simulink library "Crazyflie_Library"  (R2019a)
settings: Solver=VariableStepAuto  StartTime=0.0  StopTime=10.0  RelTol=1e-3
values from neighbouring files (symbols this model uses):
  DeePC_param = evalin('base', 'DeePC_param')    [DeePC_Optimizer_osqp.m]
  param = evalin('base', 'param')    [DeePC_Optimizer_osqp.m]    (also in DeePC_main.m = load_crazyflie_parameters(i_aux))
undefined symbols (not defined in the file or in its folder): DiscIntNeverNeededParam
libraries: simulink x3, $bdroot x3
(part 2 of 2)

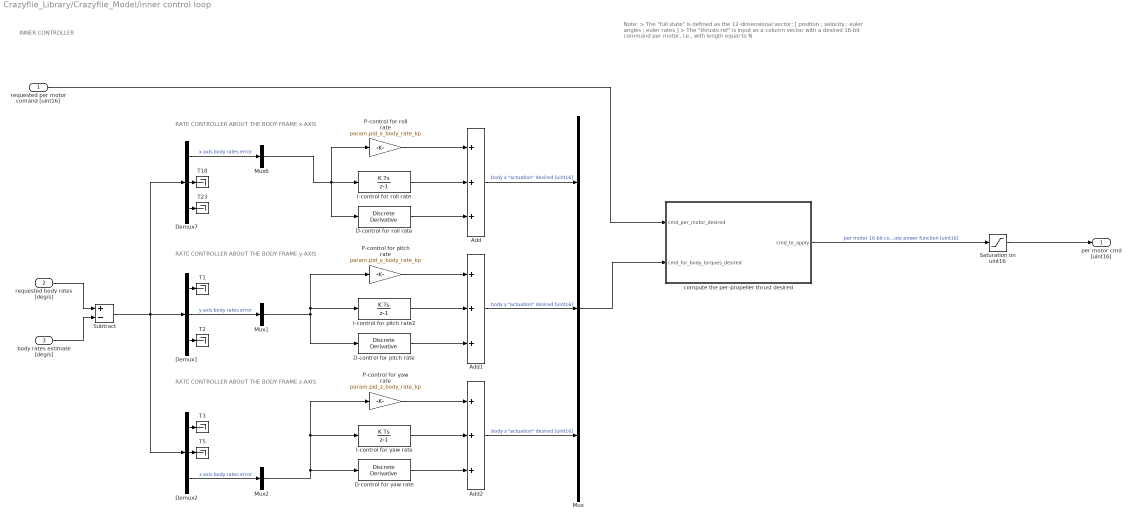
== system Crazyflie_Library/Crazyflie_Model/inner control loop ==
  note: RATE CONTROLLER ABOUT THE BODY FRAME z-AXIS
  note: RATE CONTROLLER ABOUT THE BODY FRAME y-AXIS
  note: RATE CONTROLLER ABOUT THE BODY FRAME x-AXIS
  note: INNER CONTROLLER
  note: Note:
      | > The "full state" is defined as the 12-dimensional vector:
      | [ position ; velocity ; euler angles ; euler rates ]
      | > The "thrusts ref" is input as a column vector with a desired
      | 16-bit command per motor, i.e., with length equal to N
  requested per motor comand [uint16] : Inport
  requested body rates [deg/s] : Inport  Port=2
  body rates estimate [deg/s] : Inport  Port=3
  Add : Sum  Inputs=+++
  Add1 : Sum  Inputs=+++
  Add2 : Sum  Inputs=+++
  D-control for pitch rate : simulink/Discrete/Discrete Derivative  gainval=param.pid_y_body_rate_kd  ICPrevScaledInput=0.0  OutMin=[]  OutMax=[]  OutDataType=fixdt(1, 16)  OutScaling=2^-10  DoSatur=off
  D-control for roll rate : simulink/Discrete/Discrete Derivative  gainval=param.pid_x_body_rate_kd  ICPrevScaledInput=0.0  OutMin=[]  OutMax=[]  OutDataType=fixdt(1, 16)  OutScaling=2^-10  DoSatur=off
  D-control for yaw rate : simulink/Discrete/Discrete Derivative  gainval=param.pid_z_body_rate_kd  ICPrevScaledInput=0.0  OutMin=[]  OutMax=[]  OutDataType=fixdt(1, 16)  OutScaling=2^-10  DoSatur=off
  Demux1 : Demux  Outputs=3
  Demux2 : Demux  Outputs=3
  Demux7 : Demux  Outputs=3
  I-control for pitch rate2 : DiscreteIntegrator  gainval=param.pid_y_body_rate_ki  SampleTime=-1  LimitOutput=on  UpperSaturationLimit=param.pid_y_body_rate_integrator_limit  LowerSaturationLimit=-param.pid_y_body_rate_integrator_limit  ICPrevOutput=DiscIntNeverNeededParam  ICPrevScaledInput=DiscIntNeverNeededParam
  I-control for roll rate : DiscreteIntegrator  gainval=param.pid_x_body_rate_ki  SampleTime=-1  LimitOutput=on  UpperSaturationLimit=param.pid_x_body_rate_integrator_limit  LowerSaturationLimit=-param.pid_x_body_rate_integrator_limit  ICPrevOutput=DiscIntNeverNeededParam  ICPrevScaledInput=DiscIntNeverNeededParam
  I-control for yaw rate : DiscreteIntegrator  gainval=param.pid_z_body_rate_ki  SampleTime=-1  LimitOutput=on  UpperSaturationLimit=param.pid_x_body_rate_integrator_limit  LowerSaturationLimit=-param.pid_x_body_rate_integrator_limit  ICPrevOutput=DiscIntNeverNeededParam  ICPrevScaledInput=DiscIntNeverNeededParam
  Mux : Mux  Inputs=3
  Mux1 : Mux  Inputs=1
  Mux2 : Mux  Inputs=1
  Mux6 : Mux  Inputs=1
  P-control for pitch rate : Gain  Gain=param.pid_y_body_rate_kp
  P-control for roll rate : Gain  Gain=param.pid_x_body_rate_kp
  P-control for yaw rate : Gain  Gain=param.pid_z_body_rate_kp
  Saturation on uint16 : Saturate  UpperLimit=param.cmd_max  LowerLimit=param.cmd_min  ZeroCross=off
  Subtract : Sum  Inputs=+-
  T{1..3,5,18,23} (6 alike) : Terminator
  compute the per-propeller thrust desired : MATLAB Function  TreatAsAtomicUnit=on
  per motor cmd [uint16] : Outport
  wires:
  compute the per-propeller thrust desired/1(cmd_to_apply) -> Saturation on uint16/1  "per motor 16-bit command after distribute power function [uint16]"
  body rates estimate [deg/s]/1 -> Subtract/2
  requested per motor comand [uint16]/1 -> compute the per-propeller thrust desired/1(cmd_per_motor_desired)
  requested body rates [deg/s]/1 -> Subtract/1
  Add/1 -> Mux/1  "body x \"actuation\" desired [uint16]"
  Add1/1 -> Mux/2  "body y \"actuation\" desired [uint16]"
  Add2/1 -> Mux/3  "body z \"actuation\" desired [uint16]"
  Subtract/1 -> Demux2/1, Demux1/1, Demux7/1
  Mux/1 -> compute the per-propeller thrust desired/2(cmd_for_body_torques_desired)
  Saturation on uint16/1 -> per motor cmd [uint16]/1
  Demux7/2 -> T18/1
  Mux6/1 -> P-control for roll rate/1, I-control for roll rate/1, D-control for roll rate/1
  Demux7/3 -> T23/1
  Demux7/1 -> Mux6/1  "x axis body rates error"
  Demux1/2 -> Mux1/1  "y axis body rates error"
  Demux1/3 -> T2/1
  Demux1/1 -> T1/1
  Demux2/3 -> Mux2/1  "z axis body rates error"
  Demux2/1 -> T3/1
  Mux2/1 -> I-control for yaw rate/1, P-control for yaw rate/1, D-control for yaw rate/1
  Demux2/2 -> T5/1
  P-control for roll rate/1 -> Add/1
  I-control for roll rate/1 -> Add/2
  D-control for roll rate/1 -> Add/3
  P-control for pitch rate/1 -> Add1/1
  I-control for pitch rate2/1 -> Add1/2
  D-control for pitch rate/1 -> Add1/3
  Mux1/1 -> D-control for pitch rate/1, P-control for pitch rate/1, I-control for pitch rate2/1
  D-control for yaw rate/1 -> Add2/3
  P-control for yaw rate/1 -> Add2/1
  I-control for yaw rate/1 -> Add2/2

== system Crazyflie_Library/Crazyflie_Model/N-rotor vehicle model/Full equations of motions implemented in one shot ==
  thrusts [N] : Inport
  Body rates friction matrix : Constant  Value=param.nrotor_vehicle_body_rates_friction
  Integrator5 : Integrator  InitialCondition=param.nrotor_initial_condition
  Inverse of J : Constant  Value=param.nrotor_vehicle_inertia_inverse
  Matrix describing the vehicle layout : Constant  Value=param.nrotor_vehicle_layout_true
  "Moment of inertia matrix, J" : Constant  Value=param.nrotor_vehicle_inertia
  Position friction matrix : Constant  Value=param.nrotor_vehicle_position_friction
  The full equations of motion implemented with one function : MATLAB Function  TreatAsAtomicUnit=on
  graviational constant : Constant  Value=param.g
  vehicle's mass : Constant  Value=param.nrotor_vehicle_mass_true
  full state : Outport
  body rates : Outport  Port=2
  body accellerations : Outport  Port=3
  wires:
  The full equations of motion implemented with one function/1(full_state_dot) -> Integrator5/1  "full_state_dot"
  Matrix describing the vehicle layout/1 -> The full equations of motion implemented with one function/5(layout)
  The full equations of motion implemented with one function/3(body_accel) -> body accellerations/1
  graviational constant/1 -> The full equations of motion implemented with one function/1(g)
  thrusts [N]/1 -> The full equations of motion implemented with one function/8(thrusts)
  The full equations of motion implemented with one function/2(body_rates) -> body rates/1
  Integrator5/1 -> full state/1, The full equations of motion implemented with one function/9(full_state)  "full_state"
  Inverse of J/1 -> The full equations of motion implemented with one function/4(J_inv)
  vehicle's mass/1 -> The full equations of motion implemented with one function/2(m)
  "Moment of inertia matrix, J"/1 -> The full equations of motion implemented with one function/3(J)
  Position friction matrix/1 -> The full equations of motion implemented with one function/6(pos_fric)
  Body rates friction matrix/1 -> The full equations of motion implemented with one function/7(w_fric)

== system Crazyflie_Library/Crazyflie_Model/N-rotor vehicle model/convert motor comand to thrust ==
  note: CONVERT MOTOR COMMAND AS uint16 VALUE TO THRUST IN NEWTONS
      | > Apply the following equation:
      | thust [N] = nrotor_vehicle_thrust_max * ( cmd_2_newtons_conversion_quadratic_coefficient * cmd^2 + cmd_2_newtons_conversion_linear_coefficient * cmd )
      |
      | > This sub-system acts element-wise on the input, i.e., the output is a vector of the same length as the input
  cmd [uint16] : Inport
  Add : Sum
  cmd^2 : Math  Operator=square  SaturateOnIntegerOverflow=on
  convert back to double to avoid unexpected data casting : DataTypeConversion  OutDataTypeStr=double
  linear term : Gain  Gain=param.nrotor_vehicle_thrust_max .* param.cmd_2_newtons_conversion_linear_coefficient
  quadratic term : Gain  Gain=param.nrotor_vehicle_thrust_max .* param.cmd_2_newtons_conversion_quadratic_coefficient
  thrust [N] : Outport
  wires:
  cmd^2/1 -> quadratic term/1
  quadratic term/1 -> Add/2
  linear term/1 -> Add/1
  cmd [uint16]/1 -> convert back to double to avoid unexpected data casting/1
  Add/1 -> thrust [N]/1
  convert back to double to avoid unexpected data casting/1 -> linear term/1, cmd^2/1

== matlab function Crazyflie_Library/Crazyflie_Model/Measurements/draw sample from multivariate Gaussian for gyroscope ==
  data: std_normal_rand_sample input; rand_sample output; mean_vector input; covariance_matrix_decomposition input
function rand_sample = mvn_gyroscope( std_normal_rand_sample , mean_vector , covariance_matrix_decomposition )


% Compute the multi-variate Gaussian sample from a distirbution with:
% > "mean_vector" as the mean, and
% > "covariance_matrix_decomposition" as the "square root" of the
%    covariance matrix
rand_sample = mean_vector + covariance_matrix_decomposition * std_normal_rand_sample;

== matlab function Crazyflie_Library/Crazyflie_Model/Measurements/draw sample from multivariate Gaussian for full state ==
  data: std_normal_rand_sample input; rand_sample output; mean_vector input; covariance_matrix_decomposition input
function rand_sample = mvn_full_state( std_normal_rand_sample , mean_vector , covariance_matrix_decomposition )


% Compute the multi-variate Gaussian sample from a distirbution with:
% > "mean_vector" as the mean, and
% > "covariance_matrix_decomposition" as the "square root" of the
%    covariance matrix
rand_sample = mean_vector + covariance_matrix_decomposition * std_normal_rand_sample;

== matlab function Crazyflie_Library/Crazyflie_Model/Measurements/draw sample from multivariate Gaussian for accelerometer ==
  data: std_normal_rand_sample input; rand_sample output; mean_vector input; covariance_matrix_decomposition input
function rand_sample = mvn_accelerometer( std_normal_rand_sample , mean_vector , covariance_matrix_decomposition )


% Compute the multi-variate Gaussian sample from a distirbution with:
% > "mean_vector" as the mean, and
% > "covariance_matrix_decomposition" as the "square root" of the
%    covariance matrix
rand_sample = mean_vector + covariance_matrix_decomposition * std_normal_rand_sample;

== matlab function Crazyflie_Library/Crazyflie_Model/inner control loop/compute the per-propeller thrust desired ==
  data: cmd_per_motor_desired input; cmd_for_body_torques_desired input; cmd_to_apply output
function cmd_to_apply = distribute_power( cmd_per_motor_desired , cmd_for_body_torques_desired )
% ----------------------------------------------------------------------- %
% DESCRIPTION:
% This function computes the uint16 command to apply to each motor as per
% the code that runs "on-board" on the Crazyflie's firmware
%
%
% INPUT ARGUMENTS:
%
% cmd_per_motor_desired [uint16]
% > This is a colulmn vector with length equal to the number of propellers
%   on the Crazyflie, i.e., 4, and each element represents the "baseline"
%   16-bit command that should be requested from the Crazyflie, as
%   requested by the outer loop controller.
%
% cmd_for_body_torques_desired [uint16]
% > This is the "actuation" uint16 command that comes directly from the
%   output of the Crazyflie's body rate PID controllers running in the
%   firmware. This value of command has already been adjust for the
%   dimensions of the Crazyflie, and the pattern for distributing the
%   command across the motor is provided in the exercise sheet.
%
%
% RETURN ARGUMENTS:
% % cmd_to_apply [uint16]
% > This is a colulmn vector with length equal to the number of propellers
%   on the Crazyflie, i.e., 4, and each element represents the 16-bit
%   command that will be requested from the motors
%
%
% DATA FORMAT ASSUMPTIONS:
% > the "cmd_per_motor_desired" vector is such when applied, the static
%   thrusts exert no torque about the body frame axes
%
% ----------------------------------------------------------------------- %


% Get the uint16 commands into a separate variable for each motor
cmd1 = cmd_per_motor_desired(1);
cmd2 = cmd_per_motor_desired(2);
cmd3 = cmd_per_motor_desired(3);
cmd4 = cmd_per_motor_desired(4);


% Get the desired body torques uint16 commands into a separate variable for
% the "uint16 command torque" desired about each of the body frame axes
r = cmd_for_body_torques_desired(1) / 2;
p = cmd_for_body_torques_desired(2) / 2;
y = cmd_for_body_torques_desired(3);


% These variable names have been used to partially match the code from the
% Crazyflie firmware:
% r  -  where "r" stands for roll, this is the "uint16 command torque" to
%       apply about the body-frame's x-axis, i.e., the roll-axis
% p  -  where "p" stands for pitch, this is the "uint16 command torque" to
%       apply about the body-frame's y-axis, i.e., the pitch-axis
% y  -  where "y" stands for yaw, this is the "uint16 command torque" to
%       apply about the body-frame's z-axis, i.e., the yaw-axis
%
% Note: the "/ 2" for the extraction of "r" and "p" above is simply added
% to minimic the code of the Crazyflie firmware. Presumably the Crazyflie's
% PID contollers for the body-frame roll and pitch axis are tuned with this
% factor of "/ 2" appropriately accounted for.


% Initialise the return variable "cmd_to_apply" to zeros
% > This can be required so that Simulink knows the expected size
cmd_to_apply = zeros(4,1);

% Compute the 16-bit command that should be applied from each motor as per
% the code from the Crazyflie firmware
% > For motor 1:
cmd_to_apply(1,1)  =  cmd1   - r   + p  +  y;
% > For motor 1:
cmd_to_apply(2,1)  =  cmd2   - r   - p  -  y;
% > For motor 1:
cmd_to_apply(3,1)  =  cmd3   + r   - p  +  y;
% > For motor 1:
cmd_to_apply(4,1)  =  cmd4   + r   + p  -  y;

== matlab function Crazyflie_Library/Crazyflie_Model/N-rotor vehicle model/Full equations of motions implemented in one shot/The full equations of motion implemented with one function ==
  data: g input; full_state_dot output; m input; J input; J_inv input; layout input; pos_fric input; w_fric input; thrusts input; full_state input; body_rates output; body_accel output
function [full_state_dot,body_rates,body_accel] = fcn_eom(g,m,J,J_inv,layout,pos_fric,w_fric,thrusts,full_state)
% The "full_state_dot" return argument is a column vector with 12 elements
%full_state_dot = zeros(12,1);

% ----------------------------------------------------------------------- %
% DESCRIPTION:
% This function implements the full equation of motion in one function to
% simplify the exposition.
%
%
% INPUT ARGUMENTS:
% m
% > This is the mass of the vehicle, in units of kilograms
%
% g
% > This is the acceleration due to gravity (typically 9.81), in units of
%   meters per second squared
%
% J
% > This is the moment of inertia matrix of the vehicle (it should be a
%   3-by3 matrix), the units of each element is kilogram meters squared
%
% J_inv
% > This is the inverse of the momement of inertia matrix, it is not
%   compute in this script to reduce the simulation run time slightly
%
% layout
% > This is a matrix that specifies the layout via the following format:
% nrotor_vehicle_layout = [...
%       x_1  ,  x_2  ,  ...  ,  x_{N-1}  ,  x_{N}  ;...
%       y_1  ,  y_2  ,  ...  ,  y_{N-1}  ,  y_{N}  ;...
%       c_1  ,  c_2  ,  ...  ,  c_{N-1}  ,  c_{N}   ...
%   ];
% where:
%   > x_i   is the x coordinate of propeller "i" relative to the CoG
%   > y_i   is the y coordinate of propeller "i" relative to the CoG
%   > c_i   is the thurst to torque coefficient of the propeller, with the
%           sign used to indicate the propeller's direction of rotation,
%           +ve indicates clock-wise propeller rotation.
%
% thrusts
% > This is a colulmn vector with length equal to the number of propellers
%   on the N-rotor vehicle, and each element represents the thrust force in
%   Newtons being produced by the respective propeller
%
% full_state
% > This is a vector of length 12 and is order as:
%   full_state[1:3]     the x,y,z posiiton of the body frame origin
%                       expressed in inertial frame coordinates, in units
%                       of [meters].
%
%   full_state[4:6]     the x,y,z linear velocity of the body frame origin
%                       expressed in inertial frame coordinates, in units
%                       of [meters per second].
%
%   full_state[7:9]     the roll, pitch, and yaw intrinsic Euler angles
%                       respectively, in units of [radians].
%
%   full_state[10:12]   the angular velocity of the roll, pitch, and yaw
%                       intrinsic Euler angles respectively, in units of
%                       [radians per second].
%
% pos_fric
% > This is a 3x3 matrix with friction coefficients for x, y, and z
% velocities. It implements a primitive linear friction model.
%
% w_fric
% > This is a 3x3 matrix with friction coefficients for body rates. It
% implements a primitive linear friction model.
%
%
% RETURN ARGUMENTS:
% full_state_dot
% > This is a vector of length 12 and is ordered as:
%   full_state_dot[1:3]
%      - This is position dot and is taken directly as full_state[4:6]
%
%   full_state_dot[4:6]
%      - This is the position double dot and is computed using the equation
%        of motion for transaltion, it has units of [meters per second
%        squared]
%
%   full_state_dot[7:9]
%      - This is the angular velocity of the intrinsic Euler angles and is
%        taken directly as full_state[10:12]
%
%   full_state_dot[10:12]
%      - This is the angular accelerations of the intrinsic Euler angles
%        and is computed using the equation of motion for Euler angle
%        rotations, it has units of [radians per second squared]
%
% body_rates
% > This is a vector of length 3, each element represents the angular
%   velocity of the body frame as measured about the body frame's
%   coordinate axes, i.e., this is exactly what is measured by a typical
%   strap-down Inertial Measurement Unit (IMU) that is attached to the body
%   of most all flying vehicles. It is computed directly from the "psi_dot"
%   by that is extracted from the "full_state" by applying the
%   transformation matrix "T". It has units of [radians per second];
%
% body_accel
% > This is a vector of length 3, each element represents the linear
%   accelerations of the body frame as measured along the body frame's
%   coordinate axes, i.e., this is exctly what is measured by a typical
%   strap-down Inertial Measurement Unit (IMU). It is computed directly
%   from the "pos_double_dot" by applying the rotation matrix from inertial
%   to body frame. It has units of [meters per second squared].
%
%
% DATA FORMAT ASSUMPTIONS:
% > That the "p" is ordered as:
%   p = [ x ; y ; z ];
% > And equivalently that the "psi_dot" is ordered as:
%   p_dot = [ x_dot ; y_dot ; z_dot ];
% > That the "psi" is ordered as:
%   psi = [ roll ; pitch ; yaw ];
% > And equivalently that the "psi_dot" is ordered as:
%   psi_dot = [ roll_dot ; pitch_dot ; yaw_dot ];
% > That the "w" is ordered as:
%   w = [ w_x ; w_y ; w_z ];
%
% ----------------------------------------------------------------------- %


% Extract the components of the full state
%pos      =  full_state(1:3);
pos_dot  =  full_state(4:6);
psi      =  full_state(7:9);
psi_dot  =  full_state(10:12);


% Extract each Euler angles
r  =  psi(1);  % Roll
p  =  psi(2);  % Pitch
y  =  psi(3);  % Yaw


% Extract each Euler anglular rates
rdot  =  psi_dot(1);  % Roll  angular velocity
pdot  =  psi_dot(2);  % Pitch angular velocity
%ydot  =  psi_dot(3); % Yaw   angular velocity, not needed


% Compute the rotation matrix from body frame to inertial frame:
R_B2I = [...
         cos(y)*cos(p)  ,  cos(y)*sin(p)*sin(r)-sin(y)*cos(r)  ,  cos(y)*sin(p)*cos(r)+sin(y)*sin(r)  ;...
         sin(y)*cos(p)  ,  sin(y)*sin(p)*sin(r)+cos(y)*cos(r)  ,  sin(y)*sin(p)*cos(r)-cos(y)*sin(r)  ;...
        -sin(p)         ,  cos(p)*sin(r)                       ,  cos(p)*cos(r)                        ...
    ];


% Compute the T matrix:
T = [...
        1  ,  0       ,  -sin(p)         ;...
        0  ,  cos(r)  ,   sin(r)*cos(p)  ;...
        0  , -sin(r)  ,   cos(r)*cos(p)   ...
    ];


% Compute the T inverse matrix:
T_inv = [...
        1  ,  sin(r)*tan(p)  ,   cos(r)*tan(p)  ;...
        0  ,  cos(r)         ,  -sin(r)         ;...
        0  ,  sin(r)*sec(p)  ,   cos(r)*sec(p)   ...
    ];


% Compute the time derivative of the T matrix:
T_dot = [...
        0  ,   0            ,  -pdot*cos(p)                            ;...
        0  ,  -rdot*sin(r)  ,   rdot*cos(r)*cos(p)-pdot*sin(r)*sin(p)  ;...
        0  ,  -rdot*cos(r)  ,  -rdot*sin(r)*cos(p)-pdot*cos(r)*sin(p)   ...
    ];


% Implement the equation of motion for translation
pos_double_dot = (1/m) .* ( R_B2I * [0;0;sum(thrusts(:))] ) + [0;0;-g]...
    - pos_fric * pos_dot;


% Compute the body rates from the Euler angluar rates
w = T * psi_dot;


% Implement the equation of motion for body frame rotations
w_dot = J_inv * ( [layout(2,:);-layout(1,:);layout(3,:)] * thrusts - cross( w , J*w ) )...
    - w_fric * w;

% Implement the equation of motion for Euler angle rotations
psi_double_dot = T_inv * ( w_dot - T_dot * psi_dot );


% Put together the "full_state_dot" return variable
full_state_dot = [...
        pos_dot ;...
        pos_double_dot ;...
        psi_dot ;...
        psi_double_dot ...
    ];


% Put together the "body_rates" return variable
body_rates = w;


% Finally compute the accelerations in the body frame
% > by "simply" rotating the inertial frame linear accelerations, i.e.,
%   "pos_double_dot", from the inertial frame into the body frame
body_accel = transpose(R_B2I) * pos_double_dot - cross(w, transpose(R_B2I) * pos_dot);


end

== matlab function Crazyflie_Library/LQR_Controller/MATLAB Function ==
  data: current_yaw input; xy_error_in_inertial_frame input; xy_error_in_body_frame output
function xy_error_in_body_frame = rotate_xy_intertial_to_body( current_yaw , xy_error_in_inertial_frame )
% ----------------------------------------------------------------------- %
% DESCRIPTION:
% This function rotates an (x,y) coordainte and (x_dot,y_dot) velocity
% vector from the interial frame into (approximately) the body frame. The
% approximate is because the rotation into the body frame is only based on
% the current yaw of the vehicle and assumes that roll and pitch are zero.
%
%
% INPUT ARGUMENTS:
% current_yaw
% > The intrinsic Euler yaw angle, in radians
%
% xy_error_in_inertial_frame [m;m;m/s;m/s]
% > The measurement of (x,y) position and velocities in the inertial frame
%
%
% RETURN ARGUMENTS:
% xy_error_in_body_frame
% > The measurement of (x,y) position and velocities rotated into the body
%   frame
%
%
% ----------------------------------------------------------------------- %


% Extract the inertial position and velocities
x_I      =  xy_error_in_inertial_frame(1);
y_I      =  xy_error_in_inertial_frame(2);
xdot_I   =  xy_error_in_inertial_frame(3);
ydot_I   =  xy_error_in_inertial_frame(4);

% Save some computation
cosYaw = cos(current_yaw);
sinYaw = sin(current_yaw);

% Initialise the return variable "xy_error_in_body_frame" to zeros
% > This can be required so that Simulink knows the expected size
xy_error_in_body_frame = zeros(4,1);


% Rotate the inertial POSITIONS into the body frame
% > For computing x in the body frame
xy_error_in_body_frame(1,1) =  x_I * cosYaw + y_I * sinYaw;
% > For computing y in the body frame
xy_error_in_body_frame(2,1) =  y_I * cosYaw - x_I * sinYaw;


% Rotate the inertial VELOCITIES into the body frame
% > For computing xdot in the body frame
xy_error_in_body_frame(3,1) =  xdot_I * cosYaw + ydot_I * sinYaw;
% > For computing ydot in the body frame
xy_error_in_body_frame(4,1) =  ydot_I * cosYaw - xdot_I * sinYaw;

== matlab function Crazyflie_Library/Crazyflie_Linearized_Model/Measurements/draw sample from multivariate Gaussian for full state ==
  data: std_normal_rand_sample input; rand_sample output; mean_vector input; covariance_matrix_decomposition input
function rand_sample = mvn_full_state( std_normal_rand_sample , mean_vector , covariance_matrix_decomposition )


% Compute the multi-variate Gaussian sample from a distirbution with:
% > "mean_vector" as the mean, and
% > "covariance_matrix_decomposition" as the "square root" of the
%    covariance matrix
rand_sample = mean_vector + covariance_matrix_decomposition * std_normal_rand_sample;

== matlab function Crazyflie_Library/Crazyflie_Linearized_Model_w_Gravity/Measurements/draw sample from multivariate Gaussian for full state ==
  data: std_normal_rand_sample input; rand_sample output; mean_vector input; covariance_matrix_decomposition input
function rand_sample = mvn_full_state( std_normal_rand_sample , mean_vector , covariance_matrix_decomposition )


% Compute the multi-variate Gaussian sample from a distirbution with:
% > "mean_vector" as the mean, and
% > "covariance_matrix_decomposition" as the "square root" of the
%    covariance matrix
rand_sample = mean_vector + covariance_matrix_decomposition * std_normal_rand_sample;
